simulink model "mantran_mdl_demo_v14"  (Simulink 7.0)
settings: Solver=ode3  StartTime=0.0  StopTime=100  FixedStep=0.001  RelTol=1e-3
PreLoadFcn:
  | eng_mdl_demo_v14_setup
InitFcn:
  | eng_mdl_demo_v14_setup
undefined symbols (not defined in the file or in its folder): notex
libraries: hil14_mdl_lib x1, ni_annotations_lib x1
CloseFcn:
  | eng_mdl_demo_v14_close
settings Model: Creator=Eric Bradley  LastModifiedBy=Eric Bradley
settings OptimizationCC: SimCompilerOptimization=On
settings DebuggingCC: InheritedTsInSrcMsg=none  ParameterPrecisionLossMsg=none
settings RTWCC: SystemTargetFile=NIVeriStand.tlc  TemplateMakefile=NIVeriStand_vc.tmf  Description=NI VeriStand Real-Time Target for Release 2007b or later  ProcessScript=NIVeriStand_make_rtw_hook
settings STFCustomTargetCC: GenFloatMathFcnCalls=ANSI_C  MatFileLogging=on  SystemTargetFile=NIVeriStand.tlc
settings CustomProperty: Value=on
settings EnumStrPairs: String=Default

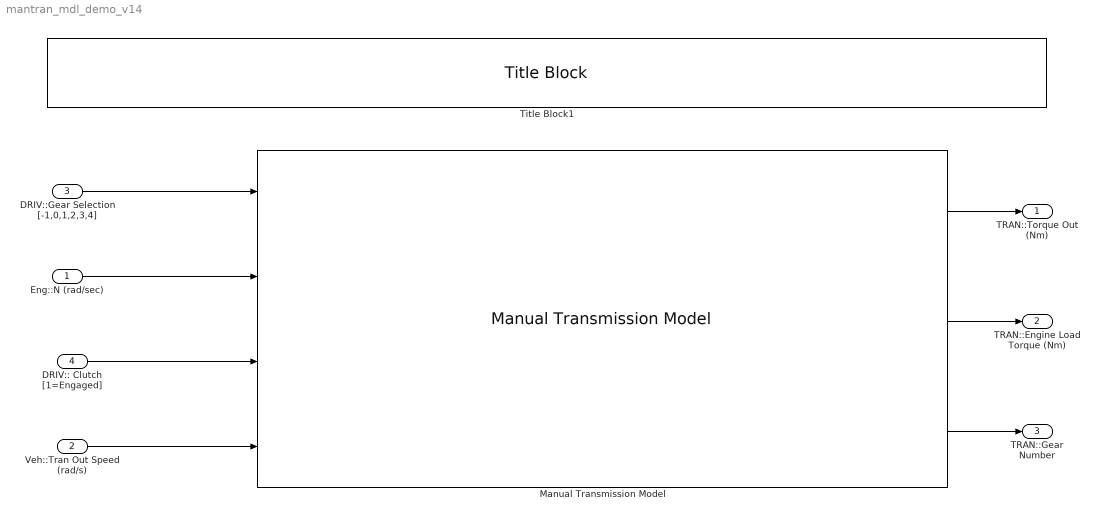
== system mantran_mdl_demo_v14 ==
  Eng::N (rad/sec) : Inport  OutDataType=sfix(16)  OutScaling=2^0
  Veh::Tran Out Speed (rad/s) : Inport  Port=2  OutDataType=sfix(16)  OutScaling=2^0
  DRIV::Gear Selection [-1,0,1,2,3,4] : Inport  Port=3  OutDataType=sfix(16)  OutScaling=2^0
  DRIV:: Clutch [1=Engaged] : Inport  Port=4  OutDataType=sfix(16)  OutScaling=2^0
  Manual Transmission Model : hil14_mdl_lib/Manual Transmission Model  SystemSampleTime=-1  iname='Manual_Transmission.png'  scale=0.55
  Title Block1 : ni_annotations_lib/Title Block  SystemSampleTime=-1  tx_title=notex(get_param(gcs,'Name'))
  TRAN::Torque Out (Nm) : Outport  OutDataType=sfix(16)  OutScaling=2^0
  TRAN::Engine Load Torque (Nm) : Outport  Port=2  OutDataType=sfix(16)  OutScaling=2^0
  TRAN::Gear Number : Outport  Port=3  OutDataType=sfix(16)  OutScaling=2^0
  wires:
  Eng::N (rad/sec)/1 -> Manual Transmission Model/2
  Veh::Tran Out Speed (rad/s)/1 -> Manual Transmission Model/4
  Manual Transmission Model/1 -> TRAN::Torque Out (Nm)/1
  Manual Transmission Model/2 -> TRAN::Engine Load Torque (Nm)/1
  Manual Transmission Model/3 -> TRAN::Gear Number/1
  DRIV::Gear Selection [-1,0,1,2,3,4]/1 -> Manual Transmission Model/1
  DRIV:: Clutch [1=Engaged]/1 -> Manual Transmission Model/3
